simulink model "mpc555rt_fuelsys"  (Simulink 6.0)
settings: Solver=ode3  SolverMode=SingleTasking  StartTime=0.0  StopTime=8  FixedStep=0.01  RelTol=1e-5  AbsTol=1e-6
PreLoadFcn:
  | RTWConfigurationCB('preloadfcn', bdroot);load mpc555_fuelsysdata.mat
InitFcn:
  | % START RTW CONFIGURATION CODE %
  | RTWConfigurationCB('rtw_target_initfcn',gcs);
  | % END RTW CONFIGURATION CODE %
libraries: mpc555drivers x3, mpc555_fuelsys_project x1
CloseFcn:
  | rtwprivate ssgencode ModelCloseRequest ssdemo_pil_build
settings Model: CovMetricSettings=d  Creator=The MathWorks Inc.  LastModifiedBy=batserve  ExtModeTrigMode=oneshot  ExtModeArmWhenConnect=off  ExtModeAutoUpdateStatusClock=off  ProdHWDeviceType=Motorola PowerPC
settings DataIOCC: LimitDataPoints=off  SaveOutput=off  SaveTime=off  SignalLoggingName=sigsOut
settings OptimizationCC: BlockReduction=off  InlineParams=on  InlineInvariantSignals=off  OptimizeModelRefInitCode=on  LifeSpan=1
settings DebuggingCC: CheckExecutionContextPreStartOutputMsg=on  CheckExecutionContextRuntimeOutputMsg=on  SolverPrmCheckMsg=none  IntegerOverflowMsg=none
settings HardwareCC: ProdEndianess=BigEndian  ProdHWDeviceType=Motorola PowerPC
settings RTWCC: SystemTargetFile=mpc555rt.tlc  TemplateMakefile=mpc555rt.tmf  RetainRTWFile=on  ProcessScript=mpc555rt_make_rtw_hook
settings CodeAppCC: IgnoreCustomStorageClasses=off
settings STFCustomTargetCC: TargetFcnLib=ansi_tfl_tmw.mat  GenFloatMathFcnCalls=ANSI_C  ModelReferenceCompliant=off  CombineOutputUpdateFcns=on  ERTCustomFileBanners=on  SystemTargetFile=mpc555rt.tlc
settings ERTTargetCC: TargetFcnLib=ansi_tfl_tmw.mat  GenFloatMathFcnCalls=ANSI_C  ModelReferenceCompliant=off  SupportContinuousTime=on  SupportNonInlinedSFcns=on  RootIOFormat=Individual Arguments  ERTCustomFileTemplate=example_file_process.tlc  InitialValueSource=Model
settings CustomProperty: DataType=RTWOptions_EnumType__toolbox_rtw_targets_mpc555dk_mpc555dk_mpc555rt_MPC555_OPTIMIZATION_SWITCH  Value=speed
settings EnumStrPairs: String=speed

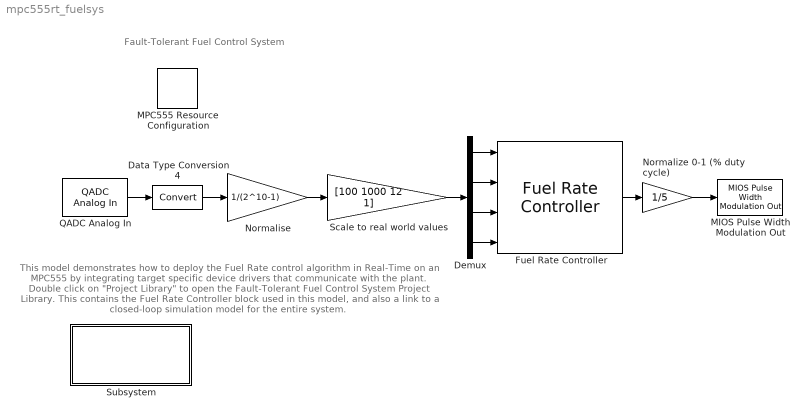
== system mpc555rt_fuelsys ==
  note: Fault-Tolerant Fuel Control System
  note: This model demonstrates how to deploy the Fuel Rate control algorithm in
      | Real-Time on an MPC555 by integrating target specific device drivers that
      | communicate with the plant.
      |
      | Double click on "Project Library" to open the Fault-Tolerant Fuel Control System
      | Project Library. This contains the Fuel Rate Controller block used in this model, and
      | also a link to a closed-loop simulation model for the entire system.
  Data Type Conversion4 : DataTypeConversion  OutDataTypeMode=double  SaturateOnIntegerOverflow=on  RndMeth=Zero
  Demux : Demux
  Fuel Rate Controller : mpc555_fuelsys_project/Fuel Rate Controller
  MIOS Pulse Width Modulation Out : mpc555drivers/Modular Input//Output System (MIOS1)/MIOS Pulse Width Modulation Out  Priority=2  module=0  timing_settings=off  period=0.0375  initpw=0.5  cp=255  pp=46875  t=-1  pol=off  trsp=off  fren=off  enablePassThru=off
  MPC555 Resource Configuration : mpc555drivers/MPC555 Resource Configuration  Tag=RTW CONFIGURATION BLOCK  oldParentName=mpc555rt_fuelsys  oldBlockName=|  defaultConfigLibrary=mpc555drivers
      | mpc555rt_fuelsys/MPC555
      | Resource
      | Configuration
  Normalise : Gain  Gain=1/(2^10-1)  SaturateOnIntegerOverflow=on
  Normalize 0-1 (% duty cycle) : Gain  Gain=1/5  SaturateOnIntegerOverflow=on
  QADC Analog In : mpc555drivers/Queued Analog-To-Digital Converter Module-64/QADC Analog In  module=A  channels=[0 1 2 3]  justification=Right-justified (unsigned)  t=.01  enablePassThru=off
  Scale to real world values : Gain  Gain=[100 1000 12 1]  SaturateOnIntegerOverflow=on
  Subsystem : Subsystem  PropExecContextAcrossSSBoundary=on
      settings: OpenFcn=mpc555_fuelsys_project
      mask Display: disp(sprintf('Project Library'));
  wires:
  QADC Analog In/1 -> Data Type Conversion4/1
  Data Type Conversion4/1 -> Normalise/1
  Normalise/1 -> Scale to real world values/1
  Scale to real world values/1 -> Demux/1
  Demux/1 -> Fuel Rate Controller/1
  Demux/2 -> Fuel Rate Controller/2
  Demux/3 -> Fuel Rate Controller/3
  Demux/4 -> Fuel Rate Controller/4
  Normalize 0-1 (% duty cycle)/1 -> MIOS Pulse Width Modulation Out/1
  Fuel Rate Controller/1 -> Normalize 0-1 (% duty cycle)/1

== system mpc555rt_fuelsys/Subsystem ==
